simulink model "week2_cruise_control_pid"  (R2018b)
settings: Solver=VariableStepAuto  StartTime=0.0  StopTime=200  RelTol=1e-3
InitFcn:
  | week2_cruise_control
undefined symbols (not defined in the file or in its folder): Kd, Ki, Kp, v_set_speed
libraries: simulink x2
settings Model: Creator=anime  LastModifiedBy=anime

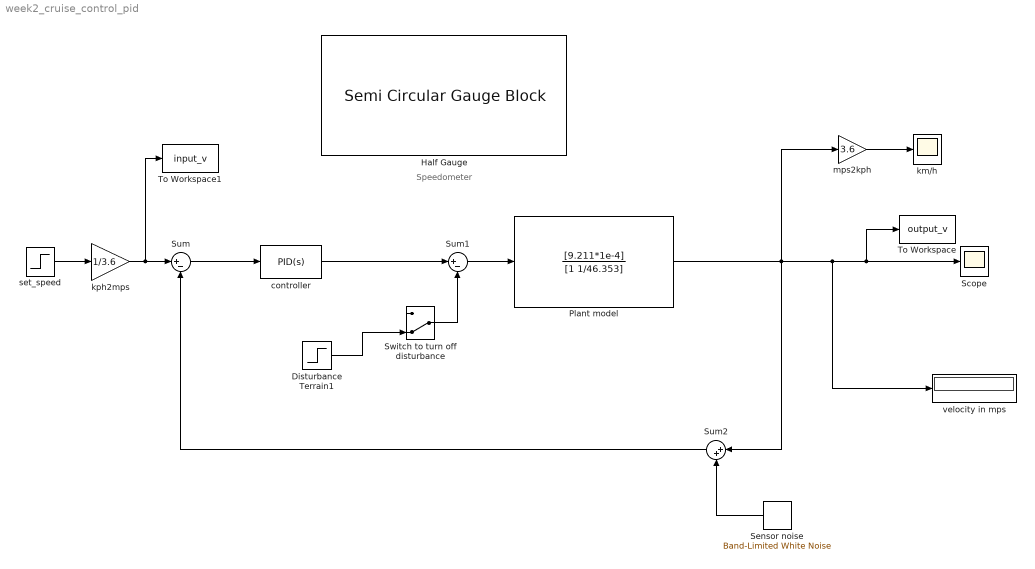
== system week2_cruise_control_pid ==
  note: Speedometer
  Disturbance Terrain1 : Step  Time=100  After=475.72*9.81*sin(pi/45)  SampleTime=0
  Half Gauge : SemiCircularGaugeBlock  WebBlockId=20  LabelPosition=Hide  ScaleMax=220
  Plant model : TransferFcn  Numerator=[9.211*1e-4]  Denominator=[1 1/46.353]
  Scope : Scope
  Sensor noise : simulink/Sources/Band-Limited White Noise  Cov=[0.001]  Ts=0.1  seed=[23341]
  Sum : Sum  Inputs=|+-
  Sum1 : Sum  Inputs=|+-
  Sum2 : Sum  Inputs=|++
  Switch to turn off disturbance : ManualSwitch  CurrentSetting=0
  To Workspace : ToWorkspace  VariableName=output_v  SaveFormat=Timeseries  SampleTime=-1
  To Workspace1 : ToWorkspace  VariableName=input_v  SaveFormat=Timeseries  SampleTime=-1
  "controller " : simulink/Continuous/PID Controller  Controller=PID  Form=Parallel  TimeDomain=Continuous-time  SampleTime=-1  IntegratorMethod=Forward Euler  FilterMethod=Forward Euler  ControllerParametersSource=internal  P=Kp  I=Ki  D=Kd  UseFilter=on  N=100  TunerSelectOption=Transfer Function Based (PID Tuner App)  InitialConditionSource=internal  InitialConditionForIntegrator=0  InitialConditionForFilter=0  DifferentiatorICPrevScaledInput=0  ExternalReset=none  TrackingMode=off  Kt=1  LimitOutput=off  UpperSaturationLimit=inf  LowerSaturationLimit=-inf  LinearizeAsGain=on  AntiWindupMode=none  Kb=1  POutMin=[]  POutMax=[]  IOutMin=[]  IOutMax=[]  DOutMin=[]  DOutMax=[]  NOutMin=[]  NOutMax=[]  SumOutMin=[]  SumOutMax=[]  SaturationOutMin=[]  SaturationOutMax=[]  PParamMin=[]  PParamMax=[]  IParamMin=[]  IParamMax=[]  DParamMin=[]  DParamMax=[]  NParamMin=[]  NParamMax=[]  KbParamMin=[]  KbParamMax=[]  KtParamMin=[]  KtParamMax=[]  KbOutMin=[]  KbOutMax=[]  KtOutMin=[]  KtOutMax=[]  IntegratorOutMin=[]  IntegratorOutMax=[]  FilterOutMin=[]  FilterOutMax=[]  SumI1OutMin=[]  SumI1OutMax=[]  SumI2OutMin=[]  SumI2OutMax=[]  SumI3OutMin=[]  SumI3OutMax=[]  SumI4OutMin=[]  SumI4OutMax=[]  SumDOutMin=[]  SumDOutMax=[]  DifferentiatorOutMin=[]  DifferentiatorOutMax=[]  FilterDiffOutCoefMin=[]  FilterDiffOutCoefMax=[]  ReciprocalOutMin=[]  ReciprocalOutMax=[]  SumDenOutMin=[]  SumDenOutMax=[]  SumNumOutMin=[]  SumNumOutMax=[]  DivideOutMin=[]  DivideOutMax=[]  IntegratorContinuousStateAttributes=''  IntegratorStateMustResolveToSignalObject=off  IntegratorRTWStateStorageClass=Auto  FilterContinuousStateAttributes=''  FilterStateMustResolveToSignalObject=off  FilterRTWStateStorageClass=Auto  ParallelPVariant=InternalParameters  IdealPVariant=Disabled  IVariant=InternalParameters  DVariant=InternalParameters  IntegratorVariant=Continuous  SatVariant=Disabled  AWVariant=Passthrough  PCopyVariant=Disabled  TRVariant=Disabled  FdbkBlocksVariant=Forward  IdealPFdbkVariant=Disabled  SatFdbkVariant=Disabled  DerivativeFilterVariant=ContFilter  NVariant=InternalParameters  NCopyVariant=Disabled  FilterICVariant=InternalICsFilter  IntegratorICVariant=InternalICs  ExternalResetVariant=Disabled  TRSumVariant=Passthrough  SumFdbkVariant=Disabled  SumVariant=Sum_PID
  km/h : Scope
  kph2mps : Gain  Gain=1/3.6
  mps2kph : Gain  Gain=3.6
  set_speed : Step  After=v_set_speed  SampleTime=0
  velocity in mps : Display
  wires:
  set_speed/1 -> kph2mps/1
  Plant model/1 -> mps2kph/1, Sum2/1, velocity in mps/1, To Workspace/1, Scope/1
  Sum/1 -> "controller "/1
  "controller "/1 -> Sum1/1
  Sum1/1 -> Plant model/1
  Switch to turn off disturbance/1 -> Sum1/2
  Disturbance Terrain1/1 -> Switch to turn off disturbance/2
  Sum2/1 -> Sum/2
  Sensor noise/1 -> Sum2/2
  mps2kph/1 -> km/h/1
  kph2mps/1 -> To Workspace1/1, Sum/1
